simulink model "SEPICPROPELLERLT"  (R2018a)
settings: Solver=ode23  StartTime=0.0  StopTime=11  RelTol=1e-3
undefined symbols (not defined in the file): R, RL
libraries: powerlib x47, powerlib_meascontrol x14, simulink x2
settings Model: Creator=dhanasekar  LastModifiedBy=AVANTHIGHA
settings SolverCC: ZeroCrossAlgorithm=Adaptive
settings DataIOCC: SaveFormat=StructureWithTime  InspectSignalLogs=on
settings OptimizationCC: LifeSpan=inf
settings DebuggingCC: MaxConsecutiveZCsMsg=none  IgnoredZcDiagnostic=none  SFExecutionAtInitializationDiag=none
settings HardwareCC: ProdBitPerSizeT=32  ProdBitPerPtrDiffT=32  ProdWordSize=32  ProdHWDeviceType=Specified
settings CodeAppCC: StateflowObjectComments=on

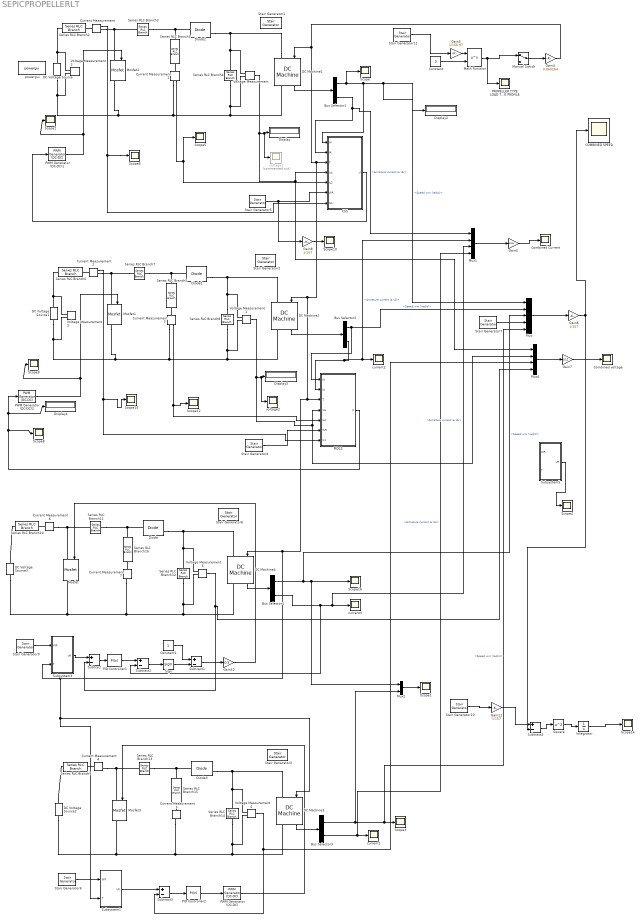
== system SEPICPROPELLERLT ==
  Bus Selector{1..4} (4 alike) : BusSelector  OutputSignals=Speed wm (rad/s),Armature current ia (A)
  COMBINED SPEED : Scope
  CSS : Subsystem
  Combined Current : Scope
  Combined voltage : Scope
  Constant : Constant  Value=3
  Constant1 : Constant
  Current Measurement{,2,4,6} (4 alike) : powerlib/Measurements/Current Measurement  PhasorSimulation=off  OutputType=Complex  PSBequivalent=0
  Current Measurement{1,3,5,7} (4 alike) : powerlib/Measurements/Current Measurement  PhasorSimulation=off  OutputType=Magnitude  PSBequivalent=0
  DC Machine{1..4} (4 alike) : powerlib/Machines/DC Machine  PresetModel=No  MechanicalLoad=Torque TL  FieldType=Permanent magnet  ShowDetailedParameters=on  MeasurementBus=off  RLa="[2.6  0.71285]"  RLf="[ 240  120]"  Laf=1.8  MachineConstant=Back-emf constant (V/rpm)  Ke=0.00525636  Kt=0.05022  J=0.0000886138  Bm=0.000096894  Tf=0  w0=0  Ifinit=1  TsPowergui=0  TsBlock=-1
      settings: SourceProductName=Simscape Electrical
  DC Voltage Source : powerlib/Electrical Sources/DC Voltage Source  Amplitude=6  Measurements=Voltage
  DC Voltage Source1 : powerlib/Electrical Sources/DC Voltage Source  Amplitude=6  Measurements=Voltage
  DC Voltage Source2 : powerlib/Electrical Sources/DC Voltage Source  Amplitude=6  Measurements=Voltage
  DC Voltage Source3 : powerlib/Electrical Sources/DC Voltage Source  Amplitude=7  Measurements=Voltage
  Diode{,1..3} (4 alike) : powerlib/Power Electronics/Diode  Ron=0.001  Lon=0  Vf=0.8  IC=0  UseSnubber=0  Rs=500  Cs=250e-9  Measurements=on
  Display{,2..4} (4 alike) : Display
  Gain10 : Gain  Gain=0.5
  Gain11 : Gain  Gain=1/157
  Gain3 : Gain  Gain=1/156.97
  Gain4 : Gain  Gain=0.060264
  Gain5 : Gain  Gain=1/1.5
  Gain6 : Gain  Gain=1/157
  Gain7 : Gain  Gain=1/12
  Gain8 : Gain  Gain=1/157
  Integrator : Integrator
  Manual Switch : ManualSwitch
  Math Function : Math  Operator=pow  SaturateOnIntegerOverflow=on
  Mosfet{,1..3} (4 alike) : powerlib/Power Electronics/Mosfet  Ron=0.1  Lon=0  Rd=0.01  Vfd=0  IC=0  Rs=1e5  Cs=inf  Measurements=on
      Mosfet1 settings: SourceProductName=Simscape Electrical
      Mosfet2 settings: SourceProductName=Simscape Electrical
  Mux : Mux  Inputs=5
  Mux1 : Mux
  Mux2 : Mux  Inputs=2
  Mux4 : Mux
  PID Controller1 : simulink/Continuous/PID Controller  Controller=PI  TimeDomain=Discrete-time  SampleTime=-1  IntegratorMethod=Forward Euler  FilterMethod=Forward Euler  Form=Parallel  UseFilter=on  ControllerParametersSource=internal  P=0.0009111115  I=1.000777777777777777  D=0.2  N=100  InitialConditionSource=internal  InitialConditionForIntegrator=0  InitialConditionForFilter=0  ExternalReset=none  LimitOutput=off  UpperSaturationLimit=inf  LowerSaturationLimit=-inf  LinearizeAsGain=on  AntiWindupMode=none  Kb=1  TrackingMode=off  Kt=1  PParamMin=[]  PParamMax=[]  IParamMin=[]  IParamMax=[]  DParamMin=[]  DParamMax=[]  NParamMin=[]  NParamMax=[]  KbParamMin=[]  KbParamMax=[]  KtParamMin=[]  KtParamMax=[]  POutMin=[]  POutMax=[]  IOutMin=[]  IOutMax=[]  DOutMin=[]  DOutMax=[]  NOutMin=[]  NOutMax=[]  KbOutMin=[]  KbOutMax=[]  KtOutMin=[]  KtOutMax=[]  IntegratorOutMin=[]  IntegratorOutMax=[]  FilterOutMin=[]  FilterOutMax=[]  SumOutMin=[]  SumOutMax=[]  SumI1OutMin=[]  SumI1OutMax=[]  SumI2OutMin=[]  SumI2OutMax=[]  SumI3OutMin=[]  SumI3OutMax=[]  SumDOutMin=[]  SumDOutMax=[]  SaturationOutMin=[]  SaturationOutMax=[]  IntegratorContinuousStateAttributes=''  IntegratorStateMustResolveToSignalObject=off  IntegratorRTWStateStorageClass=Auto  FilterContinuousStateAttributes=''  FilterStateMustResolveToSignalObject=off  FilterRTWStateStorageClass=Auto  DifferentiatorICPrevScaledInput=0  DifferentiatorOutMin=[]  DifferentiatorOutMax=[]  FilterDiffOutCoefMin=[]  FilterDiffOutCoefMax=[]  SumDenOutMin=[]  SumDenOutMax=[]  SumNumOutMin=[]  SumNumOutMax=[]  ReciprocalOutMin=[]  ReciprocalOutMax=[]  DivideOutMin=[]  DivideOutMax=[]  TunerSelectOption=Transfer Function Based (PID Tuner App)
  PID Controller2 : simulink/Continuous/PID Controller  Controller=PI  TimeDomain=Discrete-time  SampleTime=-1  IntegratorMethod=Forward Euler  FilterMethod=Forward Euler  Form=Parallel  UseFilter=on  ControllerParametersSource=internal  P=0.0000977777777777777777777777777777777777777777777777777777777777777777777777777777111115  I=1.0009999  D=0.2  N=100  InitialConditionSource=internal  InitialConditionForIntegrator=0  InitialConditionForFilter=0  ExternalReset=none  LimitOutput=off  UpperSaturationLimit=inf  LowerSaturationLimit=-inf  LinearizeAsGain=on  AntiWindupMode=none  Kb=1  TrackingMode=off  Kt=1  PParamMin=[]  PParamMax=[]  IParamMin=[]  IParamMax=[]  DParamMin=[]  DParamMax=[]  NParamMin=[]  NParamMax=[]  KbParamMin=[]  KbParamMax=[]  KtParamMin=[]  KtParamMax=[]  POutMin=[]  POutMax=[]  IOutMin=[]  IOutMax=[]  DOutMin=[]  DOutMax=[]  NOutMin=[]  NOutMax=[]  KbOutMin=[]  KbOutMax=[]  KtOutMin=[]  KtOutMax=[]  IntegratorOutMin=[]  IntegratorOutMax=[]  FilterOutMin=[]  FilterOutMax=[]  SumOutMin=[]  SumOutMax=[]  SumI1OutMin=[]  SumI1OutMax=[]  SumI2OutMin=[]  SumI2OutMax=[]  SumI3OutMin=[]  SumI3OutMax=[]  SumDOutMin=[]  SumDOutMax=[]  SaturationOutMin=[]  SaturationOutMax=[]  IntegratorContinuousStateAttributes=''  IntegratorStateMustResolveToSignalObject=off  IntegratorRTWStateStorageClass=Auto  FilterContinuousStateAttributes=''  FilterStateMustResolveToSignalObject=off  FilterRTWStateStorageClass=Auto  DifferentiatorICPrevScaledInput=0  DifferentiatorOutMin=[]  DifferentiatorOutMax=[]  FilterDiffOutCoefMin=[]  FilterDiffOutCoefMax=[]  SumDenOutMin=[]  SumDenOutMax=[]  SumNumOutMin=[]  SumNumOutMax=[]  ReciprocalOutMin=[]  ReciprocalOutMax=[]  DivideOutMin=[]  DivideOutMax=[]  TunerSelectOption=Transfer Function Based (PID Tuner App)
  PIDSS : Subsystem
  PROPELLER TYPE LOAD TORQUE PROFILE : Scope
  PWM Generator (DC-DC) : powerlib_meascontrol/Pulse & Signal Generators/PWM Generator (DC-DC)  Fsw=5000  Ts=0
  PWM Generator (DC-DC)1 : powerlib_meascontrol/Pulse & Signal Generators/PWM Generator (DC-DC)  Fsw=50000  Ts=0
      settings: SourceProductName=Simscape Electrical
  PWM Generator (DC-DC)2 : powerlib_meascontrol/Pulse & Signal Generators/PWM Generator (DC-DC)  Fsw=50000  Ts=0
      settings: SourceProductName=Simscape Electrical
  Scope{,1..6,8..10,12..14,16} (14 alike) : Scope
  Series RLC Branch{1,5..6,15..16} (5 alike) : powerlib/Elements/Series RLC Branch  LConnTagsString=__new0  RConnTagsString=__new0  BranchType=L  Resistance=RL  Inductance=0.5e-3  SetiL0=off  InitialCurrent=0  Capacitance=1e-6  Setx0=off  InitialVoltage=0  Measurements=Branch current
      settings: SourceProductName=Simscape Electrical
  Series RLC Branch10 : powerlib/Elements/Series RLC Branch  LConnTagsString=__new0  RConnTagsString=__new0  BranchType=L  Resistance=RL  Inductance=1e-3  SetiL0=off  InitialCurrent=0  Capacitance=1e-6  Setx0=off  InitialVoltage=0  Measurements=Branch current
      settings: SourceProductName=Simscape Electrical
  Series RLC Branch11 : powerlib/Elements/Series RLC Branch  LConnTagsString=__new0  RConnTagsString=__new0  BranchType=C  Resistance=R  Inductance=1e-3  SetiL0=off  InitialCurrent=0  Capacitance=10000e-6  Setx0=on  InitialVoltage=0  Measurements=Branch voltage
      settings: SourceProductName=Simscape Electrical
  Series RLC Branch{3,7,12..14} (5 alike) : powerlib/Elements/Series RLC Branch  LConnTagsString=__new0  RConnTagsString=__new0  BranchType=C  Resistance=R  Inductance=1e-3  SetiL0=off  InitialCurrent=0  Capacitance=1000e-6  Setx0=on  InitialVoltage=0  Measurements=Branch voltage
      settings: SourceProductName=Simscape Electrical
  Series RLC Branch2 : powerlib/Elements/Series RLC Branch  LConnTagsString=__new0  RConnTagsString=__new0  BranchType=L  Resistance=RL  Inductance=1e-3  SetiL0=off  InitialCurrent=0  Capacitance=1e-6  Setx0=off  InitialVoltage=0  Measurements=Branch current
      settings: SourceProductName=Simscape Electrical
  Series RLC Branch4 : powerlib/Elements/Series RLC Branch  LConnTagsString=__new0  RConnTagsString=__new0  BranchType=C  Resistance=R  Inductance=1e-3  SetiL0=off  InitialCurrent=0  Capacitance=600e-6  Setx0=on  InitialVoltage=0  Measurements=Branch voltage
      settings: SourceProductName=Simscape Electrical
  Series RLC Branch8 : powerlib/Elements/Series RLC Branch  LConnTagsString=__new0  RConnTagsString=__new0  BranchType=C  Resistance=R  Inductance=1e-3  SetiL0=off  InitialCurrent=0  Capacitance=2500e-6  Setx0=on  InitialVoltage=0  Measurements=Branch voltage
      settings: SourceProductName=Simscape Electrical
  Series RLC Branch9 : powerlib/Elements/Series RLC Branch  LConnTagsString=__new0  RConnTagsString=__new0  BranchType=L  Resistance=RL  Inductance=1e-3  SetiL0=off  InitialCurrent=0  Capacitance=1e-6  Setx0=off  InitialVoltage=0  Measurements=Branch current
      settings: SourceProductName=Simscape Electrical
  Sign : Signum
  Square : Math  Operator=square  SaturateOnIntegerOverflow=on
  Stair Generator1 : powerlib_meascontrol/Pulse & Signal Generators/Stair Generator  t=[0,4,8]  e=[0,0.0301,0.0608]  Ts=0
      settings: SourceProductName=Simscape Power Systems
  Stair Generator{4..6,9..11} (6 alike) : powerlib_meascontrol/Pulse & Signal Generators/Stair Generator  t=[0,6,10]  e=[78.5,157,94.2]  Ts=0
      settings: SourceProductName=Simscape Power Systems
  Stair Generator2 : powerlib_meascontrol/Pulse & Signal Generators/Stair Generator  t=[0,4,8]  e=[0,0.0301,0.0602]  Ts=0
      settings: SourceProductName=Simscape Power Systems
  Stair Generator3 : powerlib_meascontrol/Pulse & Signal Generators/Stair Generator  t=[0,4,8]  e=[0,0.0301,0.0602]  Ts=0
      settings: SourceProductName=Simscape Power Systems
  Stair Generator7 : powerlib_meascontrol/Pulse & Signal Generators/Stair Generator  t=[0,6,10]  e=[79.51,158,94.98]  Ts=0
      settings: SourceProductName=Simscape Power Systems
  Stair Generator8 : powerlib_meascontrol/Pulse & Signal Generators/Stair Generator  t=[0,4,8]  e=[0,0.0301,0.0602]  Ts=0
      settings: SourceProductName=Simscape Power Systems
  Subsystem1 : Subsystem
  Subsystem3 : Subsystem
  Subsystem5 : Subsystem
  Subtract{,1..4} (5 alike) : Sum  Inputs=+-
  Voltage Measurement{,1..5} (6 alike) : powerlib/Measurements/Voltage Measurement  PhasorSimulation=off  OutputType=Complex  PSBequivalent=0
  current1 : Scope
  current2 : Scope
  current3 : Scope
  powergui : powerlib/powergui  Priority=1  SimulationMode=Discrete  SampleTime=50e-6  frequency=60  Iterations=50  frequencyindice=0  Pbase=100e6  ErrMax=1e-4  UnitsV=kV  UnitsW=MW  buscounter=0  FunctionMessages=off  echomessages=off  EnableUseOfTLC=off  CurrentSourceSwitches=off  DisableSnubberDevices=off  DisableRonSwitches=off  DisableVfSwitches=off  DisplayEquations=off  SolverType=Tustin/Backward Euler (TBE)  Interpol=off  ExternalGateDelay=off  methode=off  Ts=100  x0status=blocks  SPID=on  SwTol=0  HookPort=off  RestoreLinks=warning  ResistiveCurrentMeasurement=off  Frange=[0:2:500]  Ylog=off  Xlog=on  ShowGrid=off  save=off  variable=ZData  structure=0  ZoomFFT=off  StartTime=0.0  cycles=1  DisplayStyle=1  fundamental=60  FreqAxis=off  MaxFrequency=1000  frequencyindicesteady=1  RmsSteady=1  display=off
  voltage1 : Scope  Commented=on
  voltage2 : Scope
  wires:
  Current Measurement/1 -> CSS/7(IL1), Scope6/1
  Voltage Measurement/1 -> Mux4/1, CSS/4(VA), voltage1/1, Display/1
  Current Measurement1/1 -> CSS/5(IL2), Scope5/1
  PWM Generator (DC-DC)1/1 -> Mosfet2/1, Scope2/1
  DC Machine1/1 -> Bus Selector1/1
  Bus Selector1/1 -> Scope/1, CSS/1(W), Display2/1, Mux/1  "<Speed wm (rad/s)>"
  Bus Selector1/2 -> Mux1/1, CSS/2(IA)  "<Armature current ia (A)>"
  Stair Generator5/1 -> Gain8/1, CSS/6(WR)
  CSS/1(U) -> PWM Generator (DC-DC)1/1
  DC Machine2/1 -> Bus Selector2/1
  Voltage Measurement1/1 -> voltage2/1, Display3/1, Mux4/2, PIDSS/4(VA)
  Bus Selector2/2 -> Mux1/2, current2/1, PIDSS/2(IA)  "<Armature current ia (A)>"
  PIDSS/1(U) -> Scope8/1, Display4/1, PWM Generator (DC-DC)2/1
  Current Measurement2/1 -> Scope13/1, PIDSS/7(IL1)
  Stair Generator4/1 -> PIDSS/6(WR)
  Current Measurement3/1 -> Scope12/1, PIDSS/5(IL2)
  PWM Generator (DC-DC)2/1 -> Mosfet1/1, Scope9/1
  Bus Selector2/1 -> Mux/2, PIDSS/1(W)  "<Speed wm (rad/s)>"
  Gain5/1 -> Combined Current/1
  Mux1/1 -> Gain5/1
  Mux4/1 -> Gain7/1
  Gain7/1 -> Combined voltage/1
  Mux/1 -> Gain6/1
  Gain6/1 -> Subtract4/2, COMBINED SPEED/1
  Stair Generator7/1 -> Mux/4
  Gain8/1 -> Scope10/1
  Voltage Measurement4/1 -> Mux4/3, Subtract3/2
  Integrator/1 -> Scope14/1
  Subtract/1 -> PID Controller1/1
  Square/1 -> Integrator/1
  Subtract3/1 -> PID Controller2/1
  Gain11/1 -> Subtract4/1
  Subsystem3/1(VR) -> Subtract/1
  Gain10/1 -> Mosfet/1
  PID Controller1/1 -> Subtract2/1
  Subtract2/1 -> Sign/1
  Bus Selector4/2 -> Subtract2/2, Mux1/3, current3/1  "<Armature current ia (A)>"
  Sign/1 -> Subtract1/2
  Constant1/1 -> Subtract1/1
  PID Controller2/1 -> PWM Generator (DC-DC)/1
  Bus Selector4/1 -> Mux/3, Mux2/1, Scope16/1  "<Speed wm (rad/s)>"
  Stair Generator6/1 -> Subsystem1/1(WR)
  Subsystem5/1(VR) -> Scope4/1
  Subsystem1/1(VR) -> Subtract3/1
  Mux2/1 -> Scope1/1
  Voltage Measurement5/1 -> Mux4/4, Subtract/2
  PWM Generator (DC-DC)/1 -> Mosfet3/1
  Stair Generator10/1 -> Gain11/1
  Bus Selector3/1 -> Mux2/2, Mux/5, Scope3/1  "<Speed wm (rad/s)>"
  Subtract1/1 -> Gain10/1
  Subtract4/1 -> Square/1
  Bus Selector3/2 -> Mux1/4, current1/1  "<Armature current ia (A)>"
  DC Machine4/1 -> Bus Selector4/1
  Stair Generator9/1 -> Subsystem3/1(WR)
  DC Machine3/1 -> Bus Selector3/1
  Math Function/1 -> PROPELLER TYPE LOAD TORQUE PROFILE/1, Manual Switch/1
  Gain3/1 -> Math Function/1
  Constant/1 -> Math Function/2
  Stair Generator11/1 -> Gain3/1
  Manual Switch/1 -> Gain4/1
  Gain4/1 -> Subsystem1/2(T), DC Machine3/1, Subsystem3/2(T), DC Machine4/1, PIDSS/3(T), DC Machine2/1, CSS/3(T), DC Machine1/1
  connections:
  DC Voltage Source/RConn1 -- Voltage Measurement2/LConn1 -- Series RLC Branch2/LConn1
  Current Measurement/LConn1 -- Series RLC Branch2/RConn1
  Current Measurement/RConn1 -- Mosfet2/LConn1 -- Series RLC Branch3/LConn1
  Series RLC Branch3/RConn1 -- Series RLC Branch1/LConn1 -- Diode2/LConn1
  Current Measurement1/LConn1 -- Series RLC Branch1/RConn1
  DC Machine1/LConn1 -- Diode2/RConn1 -- Voltage Measurement/LConn1 -- Series RLC Branch4/LConn1
  DC Voltage Source/LConn1 -- Voltage Measurement2/LConn2 -- Mosfet2/RConn1 -- Current Measurement1/RConn1 -- Voltage Measurement/LConn2 -- Series RLC Branch4/RConn1 -- DC Machine1/RConn1
  DC Machine2/RConn1 -- Voltage Measurement1/LConn2 -- Series RLC Branch8/RConn1 -- Current Measurement3/RConn1 -- Mosfet1/RConn1 -- DC Voltage Source1/LConn1 -- Voltage Measurement3/LConn2
  Series RLC Branch7/LConn1 -- Current Measurement2/RConn1 -- Mosfet1/LConn1
  Diode1/LConn1 -- Series RLC Branch7/RConn1 -- Series RLC Branch5/LConn1
  Series RLC Branch6/LConn1 -- DC Voltage Source1/RConn1 -- Voltage Measurement3/LConn1
  Series RLC Branch8/LConn1 -- Voltage Measurement1/LConn1 -- DC Machine2/LConn1 -- Diode1/RConn1
  Current Measurement3/LConn1 -- Series RLC Branch5/RConn1
  Current Measurement2/LConn1 -- Series RLC Branch6/RConn1
  Voltage Measurement5/LConn1 -- Series RLC Branch12/LConn1 -- DC Machine4/LConn1 -- Diode/RConn1
  Diode/LConn1 -- Series RLC Branch16/LConn1 -- Series RLC Branch11/RConn1
  Voltage Measurement4/LConn1 -- Series RLC Branch14/LConn1 -- DC Machine3/LConn1 -- Diode3/RConn1
  Mosfet3/LConn1 -- Current Measurement4/RConn1 -- Series RLC Branch13/LConn1
  Mosfet/RConn1 -- DC Voltage Source3/LConn1 -- Current Measurement7/RConn1 -- DC Machine4/RConn1 -- Voltage Measurement5/LConn2 -- Series RLC Branch12/RConn1
  Mosfet/LConn1 -- Current Measurement6/RConn1 -- Series RLC Branch11/LConn1
  Series RLC Branch14/RConn1 -- Current Measurement5/RConn1 -- DC Voltage Source2/LConn1 -- Mosfet3/RConn1 -- DC Machine3/RConn1 -- Voltage Measurement4/LConn2
  Diode3/LConn1 -- Series RLC Branch15/LConn1 -- Series RLC Branch13/RConn1
  Current Measurement7/LConn1 -- Series RLC Branch16/RConn1
  Current Measurement6/LConn1 -- Series RLC Branch10/RConn1
  Current Measurement4/LConn1 -- Series RLC Branch9/RConn1
  DC Voltage Source2/RConn1 -- Series RLC Branch9/LConn1
  Current Measurement5/LConn1 -- Series RLC Branch15/RConn1
  DC Voltage Source3/RConn1 -- Series RLC Branch10/LConn1

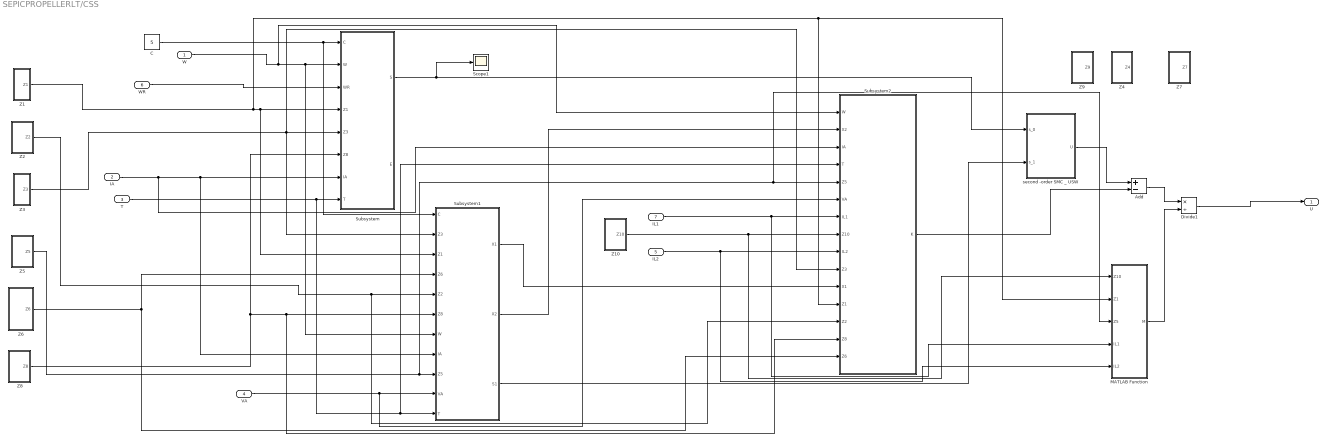
== system SEPICPROPELLERLT/CSS ==
  W : Inport
  IA : Inport  Port=2
  T : Inport  Port=3
  VA : Inport  Port=4
  IL2 : Inport  Port=5
  WR : Inport  Port=6
  IL1 : Inport  Port=7
  Add : Sum  Inputs=+-
  C : Constant  Value=5
  Divide1 : Product  Inputs=*/
  MATLAB Function : MATLAB Function  TreatAsAtomicUnit=on
  Scope1 : Scope
  Subsystem : Subsystem
  Subsystem1 : Subsystem
  Subsystem2 : Subsystem
  Z1 : Subsystem
  Z10 : Subsystem
  Z2 : Subsystem
  Z3 : Subsystem
  Z4 : Subsystem
  Z5 : Subsystem
  Z6 : Subsystem
  Z7 : Subsystem
  Z8 : Subsystem
  Z9 : Subsystem
  second -order SMC _ USW : Subsystem
  U : Outport
  wires:
  C/1 -> Subsystem1/1(C), Subsystem/1(C)
  W/1 -> Subsystem2/1(W), Subsystem1/7(W), Subsystem/2(W)
  WR/1 -> Subsystem/3(WR)
  Z1/1(Z1) -> Subsystem2/12(Z1), MATLAB Function/2(Z1), Subsystem/4(Z1), Subsystem1/3(Z1)
  Z3/1(Z3) -> Subsystem1/2(Z3), Subsystem/5(Z3), Subsystem2/10(Z3)
  Z8/1(Z8) -> Subsystem/6(Z8), Subsystem2/14(Z8), Subsystem1/6(Z8)
  IA/1 -> Subsystem2/3(IA), Subsystem1/8(IA), Subsystem/7(IA)
  T/1 -> Subsystem/8(T), Subsystem2/4(T), Subsystem1/11(T)
  Z6/1(Z6) -> Subsystem2/15(Z6), Subsystem1/4(Z6)
  Z2/1(Z2) -> Subsystem2/13(Z2), Subsystem1/5(Z2)
  Z5/1(Z5) -> MATLAB Function/3(Z5), Subsystem2/5(Z5), Subsystem1/9(Z5)
  VA/1 -> Subsystem2/6(VA), Subsystem1/10(VA)
  Subsystem1/2(X2) -> Subsystem2/2(X2)
  IL1/1 -> MATLAB Function/4(IL1), Subsystem2/7(IL1)
  Z10/1(Z10) -> MATLAB Function/1(Z10), Subsystem2/8(Z10)
  IL2/1 -> Subsystem2/9(IL2), MATLAB Function/5(IL2)
  Subsystem1/1(X1) -> Subsystem2/11(X1)
  Subsystem1/3(S1) -> second -order SMC _ USW/2(s_1)
  second -order SMC _ USW/1(U) -> Add/1
  Subsystem2/1(K) -> Add/2
  Add/1 -> Divide1/1
  MATLAB Function/1(M) -> Divide1/2
  Divide1/1 -> U/1
  Subsystem/1(S) -> Scope1/1, second -order SMC _ USW/1(s_0)

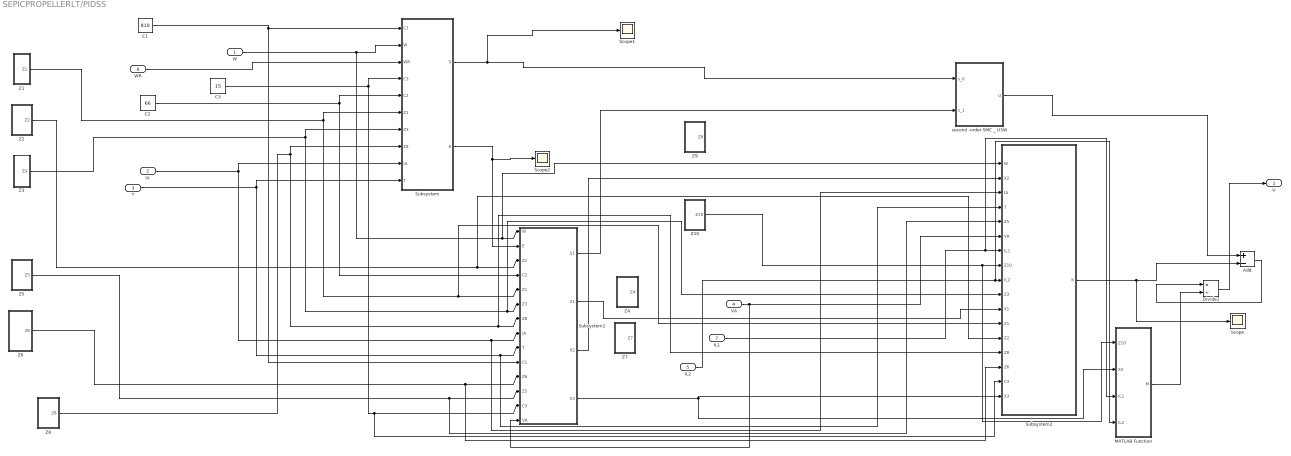
== system SEPICPROPELLERLT/PIDSS ==
  W : Inport
  IA : Inport  Port=2
  T : Inport  Port=3
  VA : Inport  Port=4
  IL2 : Inport  Port=5
  WR : Inport  Port=6
  IL1 : Inport  Port=7
  Add : Sum  Inputs=+-
  C1 : Constant  Value=810
  C2 : Constant  Value=66
  C3 : Constant  Value=15
  Divide1 : Product  Inputs=*/
  MATLAB Function : MATLAB Function  TreatAsAtomicUnit=on
  Scope : Scope
  Scope1 : Scope
  Scope2 : Scope
  Subsystem : Subsystem
  Subsystem1 : Subsystem
  Subsystem2 : Subsystem
  Z1 : Subsystem
  Z10 : Subsystem
  Z2 : Subsystem
  Z3 : Subsystem
  Z4 : Subsystem
  Z5 : Subsystem
  Z6 : Subsystem
  Z7 : Subsystem
  Z8 : Subsystem
  Z9 : Subsystem
  second -order SMC _ USW : Subsystem
  U : Outport
  wires:
  C1/1 -> Subsystem1/10(C1), Subsystem/1(C1)
  W/1 -> Subsystem2/1(W), Subsystem1/1(W), Subsystem/2(W)
  WR/1 -> Subsystem/3(WR)
  C3/1 -> Subsystem/4(C3), Subsystem2/16(C3), Subsystem1/13(C3)
  C2/1 -> Subsystem1/4(C2), Subsystem/5(C2)
  Z1/1(Z1) -> Subsystem2/12(Z1), Subsystem1/5(Z1), Subsystem/6(Z1)
  Z3/1(Z3) -> Subsystem2/10(Z3), Subsystem1/6(Z3), Subsystem/7(Z3)
  Z8/1(Z8) -> Subsystem2/14(Z8), Subsystem1/7(Z8), Subsystem/8(Z8)
  IA/1 -> Subsystem2/3(IA), Subsystem1/8(IA), Subsystem/9(IA)
  T/1 -> Subsystem2/4(T), Subsystem1/9(T), Subsystem/10(T)
  Subsystem/2(E) -> Scope2/1, Subsystem1/2(E)
  Z2/1(Z2) -> Subsystem2/13(Z2), Subsystem1/3(Z2)
  Z6/1(Z6) -> Subsystem2/15(Z6), Subsystem1/11(Z6)
  Z5/1(Z5) -> Subsystem2/5(Z5), Subsystem1/12(Z5)
  Subsystem/1(S) -> second -order SMC _ USW/1(s_0), Scope1/1
  Subsystem1/1(S1) -> second -order SMC _ USW/2(s_1)
  second -order SMC _ USW/1(U) -> Add/1
  Subsystem1/3(X2) -> Subsystem2/2(X2)
  VA/1 -> Subsystem1/14(VA), Subsystem2/6(VA)
  IL1/1 -> MATLAB Function/3(IL1), Subsystem2/7(IL1)
  IL2/1 -> MATLAB Function/4(IL2), Subsystem2/9(IL2)
  Z10/1(Z10) -> MATLAB Function/1(Z10), Subsystem2/8(Z10)
  Subsystem1/2(X1) -> Subsystem2/11(X1)
  Subsystem1/4(X3) -> MATLAB Function/2(X3), Subsystem2/17(X3)
  Subsystem2/1(K) -> Scope/1, Add/2
  Add/1 -> Divide1/1
  MATLAB Function/1(M) -> Divide1/2
  Divide1/1 -> U/1

== system SEPICPROPELLERLT/Subsystem1 ==
  WR : Inport
  T : Inport  Port=2
  A1 : Subsystem
  MATLAB Function : MATLAB Function  TreatAsAtomicUnit=on
  MATLAB Function2 : MATLAB Function  TreatAsAtomicUnit=on
  Subsystem : Subsystem
  Subsystem6 : Subsystem
  VR : Outport
  wires:
  MATLAB Function2/1(VR) -> VR/1
  Subsystem/1(A3) -> MATLAB Function/1(A3)
  A1/1(A1) -> MATLAB Function/5(A1)
  Subsystem6/1(A8) -> MATLAB Function/3(A8)
  MATLAB Function/1(IAS) -> MATLAB Function2/2(IAS)
  WR/1 -> MATLAB Function2/1(WR), MATLAB Function/2(WR)
  T/1 -> MATLAB Function/4(T)

== system SEPICPROPELLERLT/Subsystem3 ==
  WR : Inport
  T : Inport  Port=2
  A1 : Subsystem
  MATLAB Function : MATLAB Function  TreatAsAtomicUnit=on
  MATLAB Function2 : MATLAB Function  TreatAsAtomicUnit=on
  Subsystem : Subsystem
  Subsystem6 : Subsystem
  VR : Outport
  wires:
  MATLAB Function2/1(VR) -> VR/1
  Subsystem/1(A3) -> MATLAB Function/1(A3)
  A1/1(A1) -> MATLAB Function/5(A1)
  Subsystem6/1(A8) -> MATLAB Function/3(A8)
  MATLAB Function/1(IAS) -> MATLAB Function2/2(IAS)
  WR/1 -> MATLAB Function2/1(WR), MATLAB Function/2(WR)
  T/1 -> MATLAB Function/4(T)

== system SEPICPROPELLERLT/Subsystem5 ==
  WR : Inport
  T : Inport  Port=2
  A1 : Subsystem
  MATLAB Function : MATLAB Function  TreatAsAtomicUnit=on
  MATLAB Function2 : MATLAB Function  TreatAsAtomicUnit=on
  Subsystem : Subsystem
  Subsystem6 : Subsystem
  VR : Outport
  wires:
  MATLAB Function2/1(VR) -> VR/1
  Subsystem/1(A3) -> MATLAB Function/1(A3)
  A1/1(A1) -> MATLAB Function/5(A1)
  Subsystem6/1(A8) -> MATLAB Function/3(A8)
  MATLAB Function/1(IAS) -> MATLAB Function2/2(IAS)
  WR/1 -> MATLAB Function2/1(WR), MATLAB Function/2(WR)
  T/1 -> MATLAB Function/4(T)

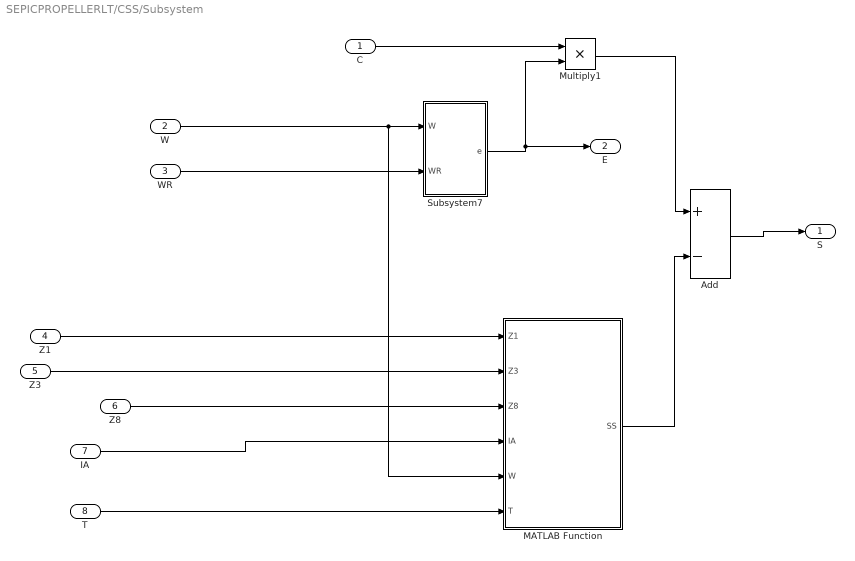
== system SEPICPROPELLERLT/CSS/Subsystem ==
  C : Inport
  W : Inport  Port=2
  WR : Inport  Port=3
  Z1 : Inport  Port=4
  Z3 : Inport  Port=5
  Z8 : Inport  Port=6
  IA : Inport  Port=7
  T : Inport  Port=8
  Add : Sum  Inputs=+-
  MATLAB Function : MATLAB Function  TreatAsAtomicUnit=on
  Multiply1 : Product
  Subsystem7 : Subsystem
  S : Outport
  E : Outport  Port=2
  wires:
  IA/1 -> MATLAB Function/4(IA)
  W/1 -> Subsystem7/1(W), MATLAB Function/5(W)
  Z8/1 -> MATLAB Function/3(Z8)
  MATLAB Function/1(SS) -> Add/2
  Multiply1/1 -> Add/1
  C/1 -> Multiply1/1
  Z1/1 -> MATLAB Function/1(Z1)
  T/1 -> MATLAB Function/6(T)
  Add/1 -> S/1
  WR/1 -> Subsystem7/2(WR)
  Z3/1 -> MATLAB Function/2(Z3)
  Subsystem7/1(e) -> E/1, Multiply1/2

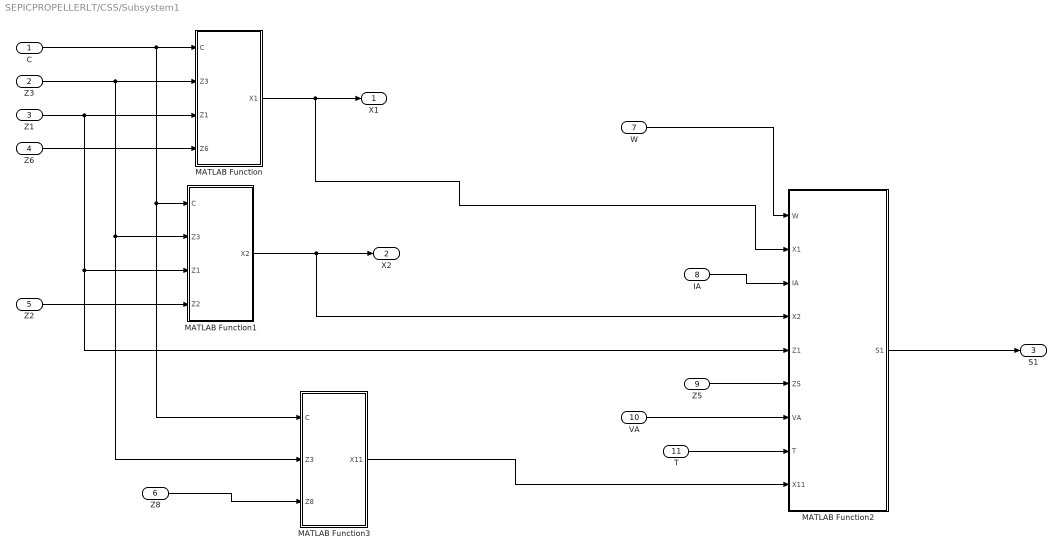
== system SEPICPROPELLERLT/CSS/Subsystem1 ==
  C : Inport
  Z3 : Inport  Port=2
  Z1 : Inport  Port=3
  Z6 : Inport  Port=4
  Z2 : Inport  Port=5
  Z8 : Inport  Port=6
  W : Inport  Port=7
  IA : Inport  Port=8
  Z5 : Inport  Port=9
  VA : Inport  Port=10
  T : Inport  Port=11
  MATLAB Function : MATLAB Function  TreatAsAtomicUnit=on
  MATLAB Function1 : MATLAB Function  TreatAsAtomicUnit=on
  MATLAB Function2 : MATLAB Function  TreatAsAtomicUnit=on
  MATLAB Function3 : MATLAB Function  TreatAsAtomicUnit=on
  X1 : Outport
  X2 : Outport  Port=2
  S1 : Outport  Port=3
  wires:
  MATLAB Function/1(X1) -> MATLAB Function2/2(X1), X1/1
  Z6/1 -> MATLAB Function/4(Z6)
  C/1 -> MATLAB Function3/1(C), MATLAB Function1/1(C), MATLAB Function/1(C)
  Z3/1 -> MATLAB Function3/2(Z3), MATLAB Function1/2(Z3), MATLAB Function/2(Z3)
  MATLAB Function1/1(X2) -> MATLAB Function2/4(X2), X2/1
  Z2/1 -> MATLAB Function1/4(Z2)
  MATLAB Function3/1(X11) -> MATLAB Function2/9(X11)
  Z8/1 -> MATLAB Function3/3(Z8)
  W/1 -> MATLAB Function2/1(W)
  IA/1 -> MATLAB Function2/3(IA)
  Z1/1 -> MATLAB Function2/5(Z1), MATLAB Function1/3(Z1), MATLAB Function/3(Z1)
  Z5/1 -> MATLAB Function2/6(Z5)
  VA/1 -> MATLAB Function2/7(VA)
  T/1 -> MATLAB Function2/8(T)
  MATLAB Function2/1(S1) -> S1/1

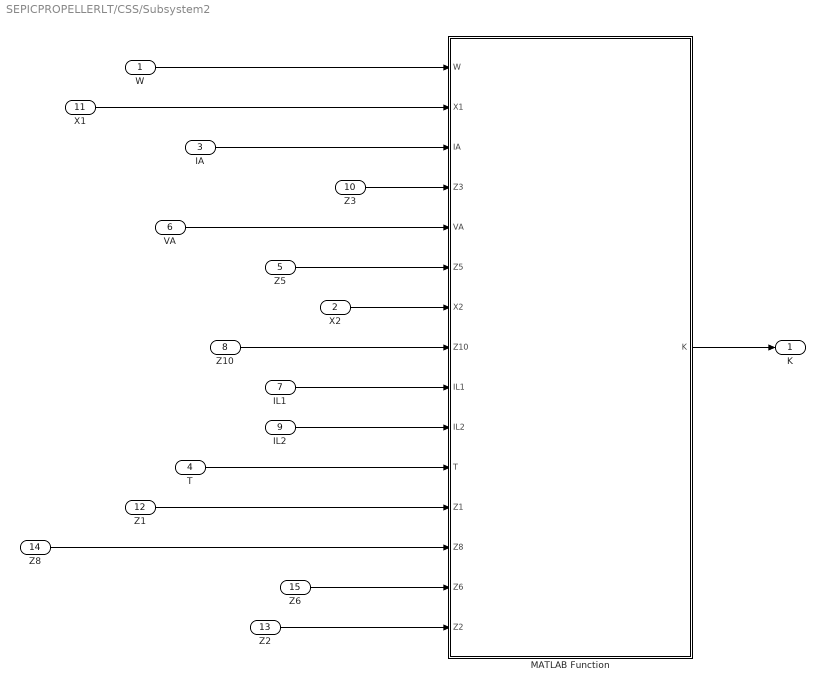
== system SEPICPROPELLERLT/CSS/Subsystem2 ==
  W : Inport
  X2 : Inport  Port=2
  IA : Inport  Port=3
  T : Inport  Port=4
  Z5 : Inport  Port=5
  VA : Inport  Port=6
  IL1 : Inport  Port=7
  Z10 : Inport  Port=8
  IL2 : Inport  Port=9
  Z3 : Inport  Port=10
  X1 : Inport  Port=11
  Z1 : Inport  Port=12
  Z2 : Inport  Port=13
  Z8 : Inport  Port=14
  Z6 : Inport  Port=15
  MATLAB Function : MATLAB Function  TreatAsAtomicUnit=on
  K : Outport
  wires:
  IA/1 -> MATLAB Function/3(IA)
  W/1 -> MATLAB Function/1(W)
  T/1 -> MATLAB Function/11(T)
  X2/1 -> MATLAB Function/7(X2)
  Z5/1 -> MATLAB Function/6(Z5)
  VA/1 -> MATLAB Function/5(VA)
  IL1/1 -> MATLAB Function/9(IL1)
  Z10/1 -> MATLAB Function/8(Z10)
  IL2/1 -> MATLAB Function/10(IL2)
  Z3/1 -> MATLAB Function/4(Z3)
  X1/1 -> MATLAB Function/2(X1)
  Z1/1 -> MATLAB Function/12(Z1)
  Z2/1 -> MATLAB Function/15(Z2)
  Z8/1 -> MATLAB Function/13(Z8)
  Z6/1 -> MATLAB Function/14(Z6)
  MATLAB Function/1(K) -> K/1

== system SEPICPROPELLERLT/CSS/Z1 ==
  Divide : Product  Inputs=*/
  J : Constant  Value=0.0000886138
  KT : Constant  Value=0.05022
  Z1 : Outport
  wires:
  KT/1 -> Divide/1
  Divide/1 -> Z1/1
  J/1 -> Divide/2

== system SEPICPROPELLERLT/CSS/Z10 ==
  1 : Constant
  C2 : Constant  Value=600e-6
  Divide1 : Product  Inputs=*/
  Z10 : Outport
  wires:
  Divide1/1 -> Z10/1
  1/1 -> Divide1/1
  C2/1 -> Divide1/2

== system SEPICPROPELLERLT/CSS/Z2 ==
  Divide : Product  Inputs=*/
  LA : Constant  Value=0.71285
  RA : Constant  Value=2.6
  Z2 : Outport
  wires:
  Divide/1 -> Z2/1
  RA/1 -> Divide/1
  LA/1 -> Divide/2

== system SEPICPROPELLERLT/CSS/Z3 ==
  B : Constant  Value=0.000096894
  Divide : Product  Inputs=*/
  J : Constant  Value=0.0000886138
  Z3 : Outport
  wires:
  B/1 -> Divide/1
  J/1 -> Divide/2
  Divide/1 -> Z3/1

== system SEPICPROPELLERLT/CSS/Z4 ==
  1 : Constant
  Divide1 : Product  Inputs=*/
  L1 : Constant  Value=10e-3
  Z4 : Outport
  wires:
  Divide1/1 -> Z4/1
  1/1 -> Divide1/1
  L1/1 -> Divide1/2

== system SEPICPROPELLERLT/CSS/Z5 ==
  1 : Constant
  Divide1 : Product  Inputs=*/
  LA1 : Constant  Value=0.71285
  Z5 : Outport
  wires:
  Divide1/1 -> Z5/1
  1/1 -> Divide1/1
  LA1/1 -> Divide1/2

== system SEPICPROPELLERLT/CSS/Z6 ==
  Divide : Product  Inputs=*/
  KE : Constant  Value=0.05022
  LA : Constant  Value=0.71285
  Z6 : Outport
  wires:
  LA/1 -> Divide/2
  KE/1 -> Divide/1
  Divide/1 -> Z6/1

== system SEPICPROPELLERLT/CSS/Z7 ==
  1 : Constant
  Divide1 : Product  Inputs=*/
  L2 : Constant  Value=5e-3
  Z7 : Outport
  wires:
  Divide1/1 -> Z7/1
  1/1 -> Divide1/1
  L2/1 -> Divide1/2

== system SEPICPROPELLERLT/CSS/Z8 ==
  1 : Constant
  Divide1 : Product  Inputs=*/
  J : Constant  Value=0.0000886138
  Z8 : Outport
  wires:
  Divide1/1 -> Z8/1
  1/1 -> Divide1/1
  J/1 -> Divide1/2

== system SEPICPROPELLERLT/CSS/Z9 ==
  1 : Constant
  C1 : Constant  Value=10e-6
  Divide1 : Product  Inputs=*/
  Z9 : Outport
  wires:
  Divide1/1 -> Z9/1
  1/1 -> Divide1/1
  C1/1 -> Divide1/2

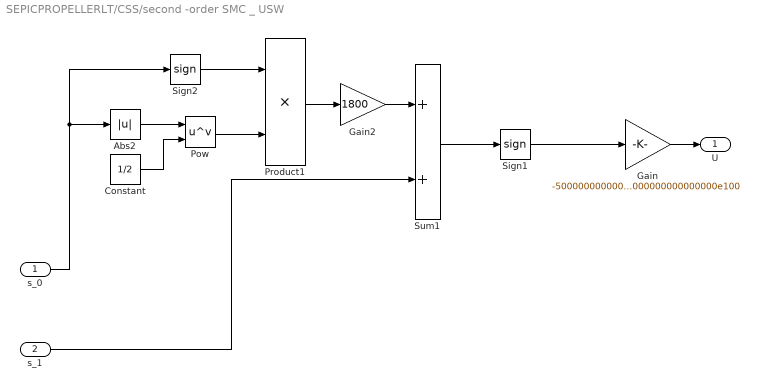
== system SEPICPROPELLERLT/CSS/second -order SMC _ USW ==
  s_0 : Inport
  s_1 : Inport  Port=2
  Abs2 : Abs
  Constant : Constant  Value=1/2
  Gain : Gain  Gain=-500000000000000000000000000000e100
  Gain2 : Gain  Gain=1800
  Pow : Math  Operator=pow  RndMeth=Zero  SaturateOnIntegerOverflow=on
  Product1 : Product
  Sign1 : Signum
  Sign2 : Signum
  Sum1 : Sum
  U : Outport
  wires:
  Gain/1 -> U/1
  s_0/1 -> Sign2/1, Abs2/1
  s_1/1 -> Sum1/2
  Sum1/1 -> Sign1/1
  Gain2/1 -> Sum1/1
  Product1/1 -> Gain2/1
  Abs2/1 -> Pow/1
  Pow/1 -> Product1/2
  Sign2/1 -> Product1/1
  Constant/1 -> Pow/2
  Sign1/1 -> Gain/1

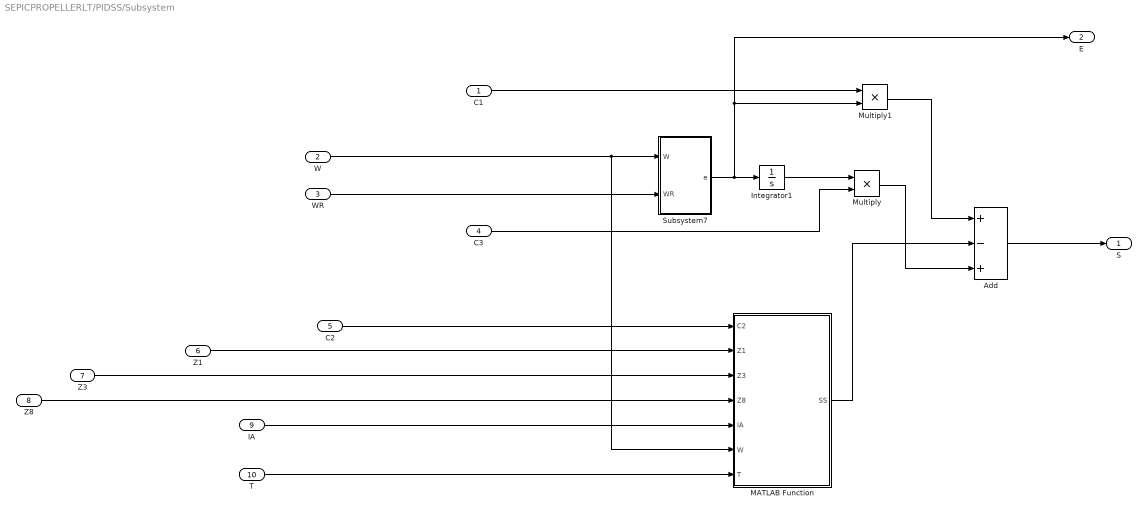
== system SEPICPROPELLERLT/PIDSS/Subsystem ==
  C1 : Inport
  W : Inport  Port=2
  WR : Inport  Port=3
  C3 : Inport  Port=4
  C2 : Inport  Port=5
  Z1 : Inport  Port=6
  Z3 : Inport  Port=7
  Z8 : Inport  Port=8
  IA : Inport  Port=9
  T : Inport  Port=10
  Add : Sum  Inputs=+-+
  Integrator1 : Integrator
  MATLAB Function : MATLAB Function  TreatAsAtomicUnit=on
  Multiply : Product
  Multiply1 : Product
  Subsystem7 : Subsystem
  S : Outport
  E : Outport  Port=2
  wires:
  IA/1 -> MATLAB Function/5(IA)
  W/1 -> MATLAB Function/6(W), Subsystem7/1(W)
  Z8/1 -> MATLAB Function/4(Z8)
  Multiply/1 -> Add/3
  MATLAB Function/1(SS) -> Add/2
  Subsystem7/1(e) -> E/1, Multiply1/2, Integrator1/1
  Multiply1/1 -> Add/1
  C1/1 -> Multiply1/1
  Z1/1 -> MATLAB Function/2(Z1)
  Integrator1/1 -> Multiply/1
  C2/1 -> MATLAB Function/1(C2)
  T/1 -> MATLAB Function/7(T)
  Add/1 -> S/1
  C3/1 -> Multiply/2
  WR/1 -> Subsystem7/2(WR)
  Z3/1 -> MATLAB Function/3(Z3)

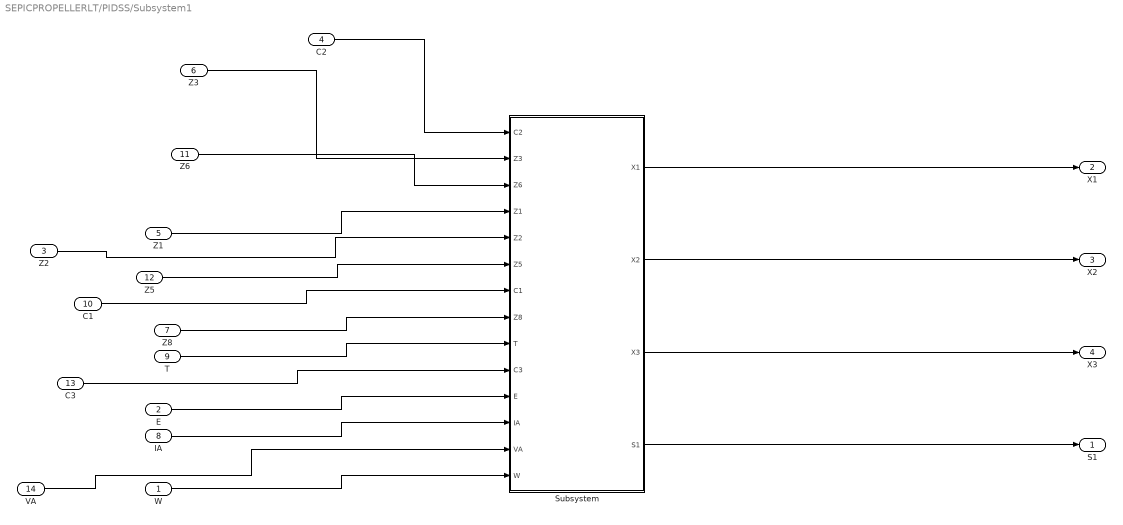
== system SEPICPROPELLERLT/PIDSS/Subsystem1 ==
  W : Inport
  E : Inport  Port=2
  Z2 : Inport  Port=3
  C2 : Inport  Port=4
  Z1 : Inport  Port=5
  Z3 : Inport  Port=6
  Z8 : Inport  Port=7
  IA : Inport  Port=8
  T : Inport  Port=9
  C1 : Inport  Port=10
  Z6 : Inport  Port=11
  Z5 : Inport  Port=12
  C3 : Inport  Port=13
  VA : Inport  Port=14
  Subsystem : Subsystem
  S1 : Outport
  X1 : Outport  Port=2
  X2 : Outport  Port=3
  X3 : Outport  Port=4
  wires:
  Subsystem/4(S1) -> S1/1
  Subsystem/1(X1) -> X1/1
  Subsystem/3(X3) -> X3/1
  Subsystem/2(X2) -> X2/1
  W/1 -> Subsystem/14(W)
  T/1 -> Subsystem/9(T)
  IA/1 -> Subsystem/12(IA)
  E/1 -> Subsystem/11(E)
  C2/1 -> Subsystem/1(C2)
  Z3/1 -> Subsystem/2(Z3)
  Z8/1 -> Subsystem/8(Z8)
  Z1/1 -> Subsystem/4(Z1)
  Z5/1 -> Subsystem/6(Z5)
  Z6/1 -> Subsystem/3(Z6)
  Z2/1 -> Subsystem/5(Z2)
  C1/1 -> Subsystem/7(C1)
  C3/1 -> Subsystem/10(C3)
  VA/1 -> Subsystem/13(VA)

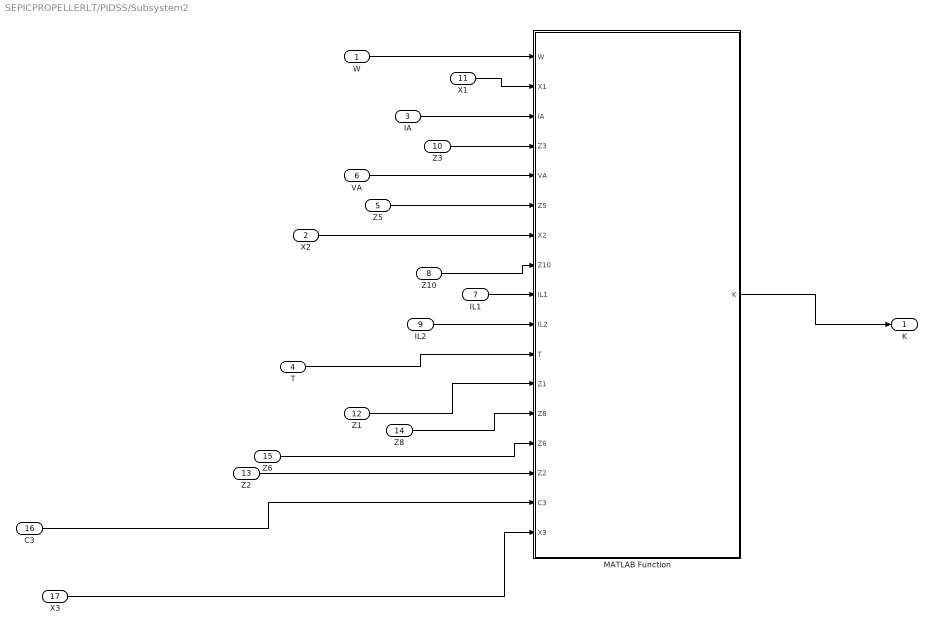
== system SEPICPROPELLERLT/PIDSS/Subsystem2 ==
  W : Inport
  X2 : Inport  Port=2
  IA : Inport  Port=3
  T : Inport  Port=4
  Z5 : Inport  Port=5
  VA : Inport  Port=6
  IL1 : Inport  Port=7
  Z10 : Inport  Port=8
  IL2 : Inport  Port=9
  Z3 : Inport  Port=10
  X1 : Inport  Port=11
  Z1 : Inport  Port=12
  Z2 : Inport  Port=13
  Z8 : Inport  Port=14
  Z6 : Inport  Port=15
  C3 : Inport  Port=16
  X3 : Inport  Port=17
  MATLAB Function : MATLAB Function  TreatAsAtomicUnit=on
  K : Outport
  wires:
  IA/1 -> MATLAB Function/3(IA)
  W/1 -> MATLAB Function/1(W)
  T/1 -> MATLAB Function/11(T)
  X2/1 -> MATLAB Function/7(X2)
  Z5/1 -> MATLAB Function/6(Z5)
  VA/1 -> MATLAB Function/5(VA)
  IL1/1 -> MATLAB Function/9(IL1)
  Z10/1 -> MATLAB Function/8(Z10)
  IL2/1 -> MATLAB Function/10(IL2)
  Z3/1 -> MATLAB Function/4(Z3)
  X1/1 -> MATLAB Function/2(X1)
  Z1/1 -> MATLAB Function/12(Z1)
  Z2/1 -> MATLAB Function/15(Z2)
  Z8/1 -> MATLAB Function/13(Z8)
  Z6/1 -> MATLAB Function/14(Z6)
  C3/1 -> MATLAB Function/16(C3)
  X3/1 -> MATLAB Function/17(X3)
  MATLAB Function/1(K) -> K/1

== system SEPICPROPELLERLT/PIDSS/Z1 ==
  Divide : Product  Inputs=*/
  J : Constant  Value=0.0000886138
  KT : Constant  Value=0.05022
  Z1 : Outport
  wires:
  KT/1 -> Divide/1
  Divide/1 -> Z1/1
  J/1 -> Divide/2

== system SEPICPROPELLERLT/PIDSS/Z10 ==
  1 : Constant
  C2 : Constant  Value=2500e-6
  Divide1 : Product  Inputs=*/
  Z10 : Outport
  wires:
  Divide1/1 -> Z10/1
  1/1 -> Divide1/1
  C2/1 -> Divide1/2

== system SEPICPROPELLERLT/PIDSS/Z2 ==
  Divide : Product  Inputs=*/
  LA : Constant  Value=0.71285
  RA : Constant  Value=2.6
  Z2 : Outport
  wires:
  Divide/1 -> Z2/1
  RA/1 -> Divide/1
  LA/1 -> Divide/2

== system SEPICPROPELLERLT/PIDSS/Z3 ==
  B : Constant  Value=0.000096894
  Divide : Product  Inputs=*/
  J : Constant  Value=0.0000886138
  Z3 : Outport
  wires:
  B/1 -> Divide/1
  J/1 -> Divide/2
  Divide/1 -> Z3/1

== system SEPICPROPELLERLT/PIDSS/Z4 ==
  1 : Constant
  Divide1 : Product  Inputs=*/
  L1 : Constant  Value=10e-3
  Z4 : Outport
  wires:
  Divide1/1 -> Z4/1
  1/1 -> Divide1/1
  L1/1 -> Divide1/2

== system SEPICPROPELLERLT/PIDSS/Z5 ==
  1 : Constant
  Divide1 : Product  Inputs=*/
  LA1 : Constant  Value=0.71285
  Z5 : Outport
  wires:
  Divide1/1 -> Z5/1
  1/1 -> Divide1/1
  LA1/1 -> Divide1/2

== system SEPICPROPELLERLT/PIDSS/Z6 ==
  Divide : Product  Inputs=*/
  KE : Constant  Value=0.05022
  LA : Constant  Value=0.71285
  Z6 : Outport
  wires:
  LA/1 -> Divide/2
  KE/1 -> Divide/1
  Divide/1 -> Z6/1

== system SEPICPROPELLERLT/PIDSS/Z7 ==
  1 : Constant
  Divide1 : Product  Inputs=*/
  L2 : Constant  Value=5e-3
  Z7 : Outport
  wires:
  Divide1/1 -> Z7/1
  1/1 -> Divide1/1
  L2/1 -> Divide1/2

== system SEPICPROPELLERLT/PIDSS/Z8 ==
  1 : Constant
  Divide1 : Product  Inputs=*/
  J : Constant  Value=0.0000886138
  Z8 : Outport
  wires:
  Divide1/1 -> Z8/1
  1/1 -> Divide1/1
  J/1 -> Divide1/2

== system SEPICPROPELLERLT/PIDSS/Z9 ==
  1 : Constant
  C1 : Constant  Value=10e-6
  Divide1 : Product  Inputs=*/
  Z9 : Outport
  wires:
  Divide1/1 -> Z9/1
  1/1 -> Divide1/1
  C1/1 -> Divide1/2

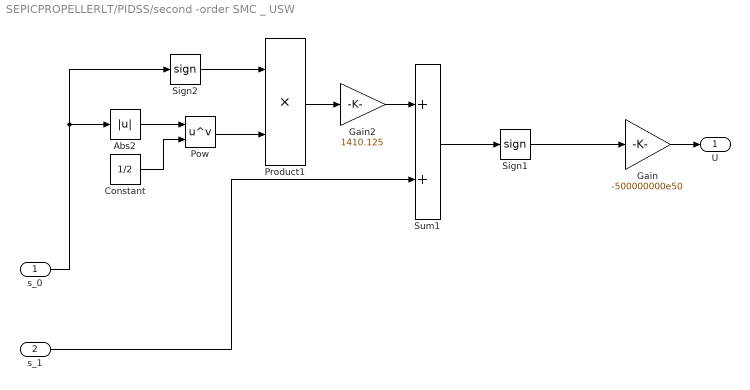
== system SEPICPROPELLERLT/PIDSS/second -order SMC _ USW ==
  s_0 : Inport
  s_1 : Inport  Port=2
  Abs2 : Abs
  Constant : Constant  Value=1/2
  Gain : Gain  Gain=-500000000e50
  Gain2 : Gain  Gain=1410.125
  Pow : Math  Operator=pow  RndMeth=Zero  SaturateOnIntegerOverflow=on
  Product1 : Product
  Sign1 : Signum
  Sign2 : Signum
  Sum1 : Sum
  U : Outport
  wires:
  Gain/1 -> U/1
  s_0/1 -> Sign2/1, Abs2/1
  s_1/1 -> Sum1/2
  Sum1/1 -> Sign1/1
  Gain2/1 -> Sum1/1
  Product1/1 -> Gain2/1
  Abs2/1 -> Pow/1
  Pow/1 -> Product1/2
  Sign2/1 -> Product1/1
  Constant/1 -> Pow/2
  Sign1/1 -> Gain/1

== system SEPICPROPELLERLT/Subsystem1/A1 ==
  Divide : Product  Inputs=*/
  J : Constant  Value=0.0000886138
  KT : Constant  Value=0.05022
  A1 : Outport
  wires:
  KT/1 -> Divide/1
  Divide/1 -> A1/1
  J/1 -> Divide/2

== system SEPICPROPELLERLT/Subsystem1/Subsystem ==
  B : Constant  Value=0.000096894
  Divide : Product  Inputs=*/
  J : Constant  Value=0.0000886138
  A3 : Outport
  wires:
  B/1 -> Divide/1
  J/1 -> Divide/2
  Divide/1 -> A3/1

== system SEPICPROPELLERLT/Subsystem1/Subsystem6 ==
  1 : Constant
  Divide1 : Product  Inputs=*/
  J : Constant  Value=0.0000886138
  A8 : Outport
  wires:
  Divide1/1 -> A8/1
  1/1 -> Divide1/1
  J/1 -> Divide1/2

== system SEPICPROPELLERLT/Subsystem3/A1 ==
  Divide : Product  Inputs=*/
  J : Constant  Value=0.0000886138
  KT : Constant  Value=0.05022
  A1 : Outport
  wires:
  KT/1 -> Divide/1
  Divide/1 -> A1/1
  J/1 -> Divide/2

== system SEPICPROPELLERLT/Subsystem3/Subsystem ==
  B : Constant  Value=0.000096894
  Divide : Product  Inputs=*/
  J : Constant  Value=0.0000886138
  A3 : Outport
  wires:
  B/1 -> Divide/1
  J/1 -> Divide/2
  Divide/1 -> A3/1

== system SEPICPROPELLERLT/Subsystem3/Subsystem6 ==
  1 : Constant
  Divide1 : Product  Inputs=*/
  J : Constant  Value=0.0000886138
  A8 : Outport
  wires:
  Divide1/1 -> A8/1
  1/1 -> Divide1/1
  J/1 -> Divide1/2

== system SEPICPROPELLERLT/Subsystem5/A1 ==
  Divide : Product  Inputs=*/
  J : Constant  Value=0.0000886138
  KT : Constant  Value=0.05022
  A1 : Outport
  wires:
  KT/1 -> Divide/1
  Divide/1 -> A1/1
  J/1 -> Divide/2

== system SEPICPROPELLERLT/Subsystem5/Subsystem ==
  B : Constant  Value=0.000096894
  Divide : Product  Inputs=*/
  J : Constant  Value=0.0000886138
  A3 : Outport
  wires:
  B/1 -> Divide/1
  J/1 -> Divide/2
  Divide/1 -> A3/1

== system SEPICPROPELLERLT/Subsystem5/Subsystem6 ==
  1 : Constant
  Divide1 : Product  Inputs=*/
  J : Constant  Value=0.0000886138
  A8 : Outport
  wires:
  Divide1/1 -> A8/1
  1/1 -> Divide1/1
  J/1 -> Divide1/2

== system SEPICPROPELLERLT/CSS/Subsystem/Subsystem7 ==
  W : Inport
  WR : Inport  Port=2
  MATLAB Function : MATLAB Function  TreatAsAtomicUnit=on
  e : Outport
  wires:
  MATLAB Function/1(e) -> e/1
  W/1 -> MATLAB Function/2(W)
  WR/1 -> MATLAB Function/1(WR)

== system SEPICPROPELLERLT/PIDSS/Subsystem/Subsystem7 ==
  W : Inport
  WR : Inport  Port=2
  MATLAB Function : MATLAB Function  TreatAsAtomicUnit=on
  e : Outport
  wires:
  MATLAB Function/1(e) -> e/1
  W/1 -> MATLAB Function/2(W)
  WR/1 -> MATLAB Function/1(WR)

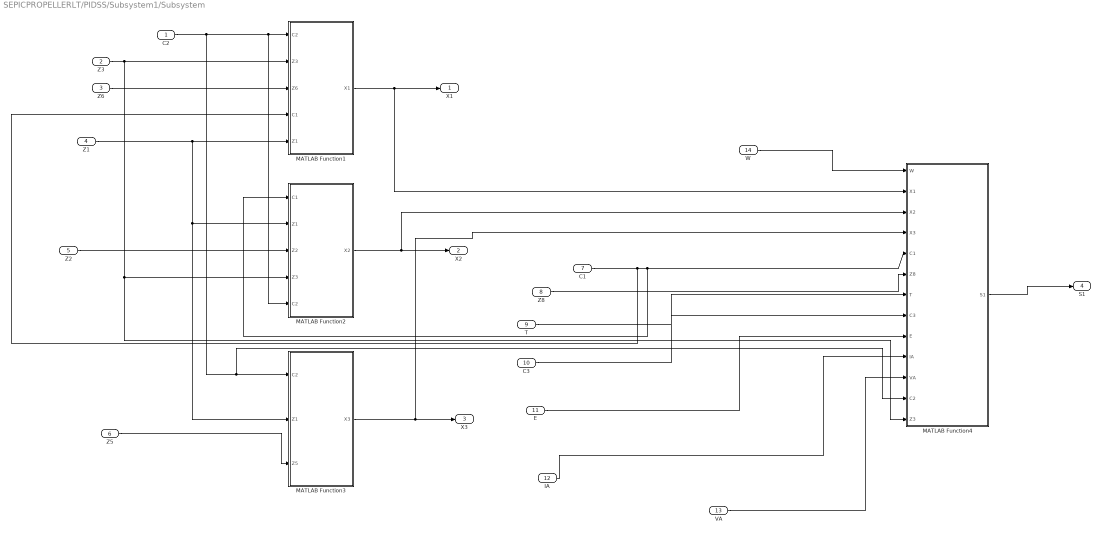
== system SEPICPROPELLERLT/PIDSS/Subsystem1/Subsystem ==
  C2 : Inport
  Z3 : Inport  Port=2
  Z6 : Inport  Port=3
  Z1 : Inport  Port=4
  Z2 : Inport  Port=5
  Z5 : Inport  Port=6
  C1 : Inport  Port=7
  Z8 : Inport  Port=8
  T : Inport  Port=9
  C3 : Inport  Port=10
  E : Inport  Port=11
  IA : Inport  Port=12
  VA : Inport  Port=13
  W : Inport  Port=14
  MATLAB Function1 : MATLAB Function  TreatAsAtomicUnit=on
  MATLAB Function2 : MATLAB Function  TreatAsAtomicUnit=on
  MATLAB Function3 : MATLAB Function  TreatAsAtomicUnit=on
  MATLAB Function4 : MATLAB Function  TreatAsAtomicUnit=on
  X1 : Outport
  X2 : Outport  Port=2
  X3 : Outport  Port=3
  S1 : Outport  Port=4
  wires:
  MATLAB Function2/1(X2) -> MATLAB Function4/3(X2), X2/1
  Z5/1 -> MATLAB Function3/3(Z5)
  C2/1 -> MATLAB Function4/12(C2), MATLAB Function3/1(C2), MATLAB Function2/5(C2), MATLAB Function1/1(C2)
  MATLAB Function3/1(X3) -> MATLAB Function4/4(X3), X3/1
  Z1/1 -> MATLAB Function2/2(Z1), MATLAB Function3/2(Z1), MATLAB Function1/5(Z1)
  Z3/1 -> MATLAB Function4/13(Z3), MATLAB Function2/4(Z3), MATLAB Function1/2(Z3)
  Z2/1 -> MATLAB Function2/3(Z2)
  Z6/1 -> MATLAB Function1/3(Z6)
  C1/1 -> MATLAB Function1/4(C1), MATLAB Function2/1(C1), MATLAB Function4/5(C1)
  MATLAB Function1/1(X1) -> MATLAB Function4/2(X1), X1/1
  Z8/1 -> MATLAB Function4/6(Z8)
  T/1 -> MATLAB Function4/7(T)
  C3/1 -> MATLAB Function4/8(C3)
  E/1 -> MATLAB Function4/9(E)
  IA/1 -> MATLAB Function4/10(IA)
  VA/1 -> MATLAB Function4/11(VA)
  MATLAB Function4/1(S1) -> S1/1
  W/1 -> MATLAB Function4/1(W)

== matlab function SEPICPROPELLERLT/CSS/Subsystem/Subsystem7/MATLAB Function ==
  data: e output; WR input; W input
function e = fcn(WR,W)

e = (WR-W);

== matlab function SEPICPROPELLERLT/CSS/Subsystem/MATLAB Function ==
  data: SS output; Z1 input; Z3 input; Z8 input; IA input; W input; T input
function SS = fcn(Z1,Z3,Z8,IA,W,T)

SS = ((Z1*IA)-(Z3*W)-(Z8*T));

== matlab function SEPICPROPELLERLT/CSS/Subsystem1/MATLAB Function ==
  data: C input; X1 output; Z3 input; Z1 input; Z6 input
function X1 = fcn(C,Z3,Z1,Z6)

X1 = ((C*Z3)+(Z1*Z6)-(Z3*Z3));

== matlab function SEPICPROPELLERLT/CSS/Subsystem1/MATLAB Function1 ==
  data: C input; X2 output; Z3 input; Z1 input; Z2 input
function X2 = fcn(C,Z3,Z1,Z2)

X2 = ((Z1*Z2)-(C*Z1)+(Z3*Z1));

== matlab function SEPICPROPELLERLT/CSS/Subsystem1/MATLAB Function2 ==
  data: W input; S1 output; X1 input; IA input; X2 input; Z1 input; Z5 input; VA input; T input; X11 input
function S1 = fcn(W,X1,IA,X2,Z1,Z5,VA,T,X11)

S1 = ((W*X1)+(IA*X2)-(Z1*Z5*VA)+(T*X11));

== matlab function SEPICPROPELLERLT/CSS/Subsystem1/MATLAB Function3 ==
  data: C input; X11 output; Z3 input; Z8 input
function X11 = fcn(C,Z3,Z8)

X11 = ((C*Z8)-(Z3*Z8));

== matlab function SEPICPROPELLERLT/CSS/Subsystem2/MATLAB Function ==
  data: W input; X1 input; IA input; Z3 input; VA input; Z5 input; X2 input; Z10 input; IL1 input; IL2 input; T input; K output; Z1 input; Z8 input; Z6 input; Z2 input
function K = fcn(W,X1,IA,Z3,VA,Z5,X2,Z10,IL1,IL2,T,Z1,Z8,Z6,Z2)

K = ((Z1*IA*X1)-(Z3*W*X1)-(Z8*T*X1)-(Z6*W*X2)-(Z2*IA*X2)+(Z5*VA*X2)-(IL1*Z1*Z5*Z10)-(IL2*Z1*Z5*Z10)+(Z10*IA*Z1*Z5));

== matlab function SEPICPROPELLERLT/CSS/MATLAB Function ==
  data: Z10 input; M output; Z1 input; Z5 input; IL1 input; IL2 input
function M = fcn(Z10,Z1,Z5,IL1,IL2)

M = ((Z10*Z1*Z5*(IL1+IL2)));

== matlab function SEPICPROPELLERLT/PIDSS/MATLAB Function ==
  data: Z10 input; M output; X3 input; IL1 input; IL2 input
function M = fcn(Z10,X3,IL1,IL2)

M = (-(Z10*X3*(IL1+IL2)));

== matlab function SEPICPROPELLERLT/PIDSS/Subsystem/MATLAB Function ==
  data: C2 input; SS output; Z1 input; Z3 input; Z8 input; IA input; W input; T input
function SS = fcn(C2,Z1,Z3,Z8,IA,W,T)

SS = (C2*((Z1*IA)-(Z3*W)-(Z8*T)));

== matlab function SEPICPROPELLERLT/PIDSS/Subsystem/Subsystem7/MATLAB Function ==
  data: e output; WR input; W input
function e = fcn(WR,W)

e = (WR-W);

== matlab function SEPICPROPELLERLT/PIDSS/Subsystem1/Subsystem/MATLAB Function1 ==
  data: X1 output; C2 input; Z3 input; Z6 input; C1 input; Z1 input
function X1 = fcn(C2,Z3,Z6,C1,Z1)

X1 = ((C1*Z3)-(C2*Z3*Z3)+(C2*Z1*Z6));

== matlab function SEPICPROPELLERLT/PIDSS/Subsystem1/Subsystem/MATLAB Function2 ==
  data: X2 output; C1 input; Z1 input; Z2 input; Z3 input; C2 input
function X2 = fcn(C1,Z1,Z2,Z3,C2)

X2 = ((C2*Z1*Z2)-(C1*Z1)+(C2*Z1*Z3));

== matlab function SEPICPROPELLERLT/PIDSS/Subsystem1/Subsystem/MATLAB Function3 ==
  data: X3 output; C2 input; Z1 input; Z5 input
function X3 = fcn(C2,Z1,Z5)

X3 = (-(C2*Z1*Z5));

== matlab function SEPICPROPELLERLT/PIDSS/Subsystem1/Subsystem/MATLAB Function4 ==
  data: S1 output; W input; X1 input; X2 input; X3 input; C1 input; Z8 input; T input; C3 input; E input; IA input; VA input; C2 input; Z3 input
function S1 = fcn(W,X1,X2,X3,C1,Z8,T,C3,E,IA,VA,C2,Z3)

S1 = ((W*X1)+(IA*X2)+(VA*X3)+(C1*Z8*T)+(C3*E)-(C2*Z3*Z8*T));

== matlab function SEPICPROPELLERLT/PIDSS/Subsystem2/MATLAB Function ==
  data: W input; X1 input; IA input; Z3 input; VA input; Z5 input; X2 input; Z10 input; IL1 input; IL2 input; T input; K output; Z1 input; Z8 input; Z6 input; Z2 input; C3 input; X3 input
function K = fcn(W,X1,IA,Z3,VA,Z5,X2,Z10,IL1,IL2,T,Z1,Z8,Z6,Z2,C3,X3)

K = ((Z1*IA*X1)-(Z3*W*X1)-(Z8*T*X1)-(Z6*W*X2)-(Z2*IA*X2)+(Z5*VA*X2)+(Z3*C3*W)-(C3*Z1*IA)+(C3*Z8*T)+(IL1*Z10*X3)+(IL2*Z10*X3)-(Z10*IA*X3));

== matlab function SEPICPROPELLERLT/Subsystem1/MATLAB Function ==
  data: A3 input; IAS output; WR input; A8 input; T input; A1 input
function IAS = fcn(A3,WR,A8,T,A1)

IAS = ((A3*WR)+(A8*T))/A1;

== matlab function SEPICPROPELLERLT/Subsystem1/MATLAB Function2 ==
  data: WR input; VR output; IAS input
function VR = fcn(WR,IAS)

VR = ((0.05022*WR)+(IAS*2.6));

== matlab function SEPICPROPELLERLT/Subsystem3/MATLAB Function ==
  data: A3 input; IAS output; WR input; A8 input; T input; A1 input
function IAS = fcn(A3,WR,A8,T,A1)

IAS = ((A3*WR)+(A8*T))/A1;

== matlab function SEPICPROPELLERLT/Subsystem3/MATLAB Function2 ==
  data: WR input; VR output; IAS input
function VR = fcn(WR,IAS)

VR = ((0.05022*WR)+(IAS*2.6));

== matlab function SEPICPROPELLERLT/Subsystem5/MATLAB Function2 ==
  data: WR input; VR output; IAS input
function VR = fcn(WR,IAS)

VR = ((0.05022*WR)+(IAS*2.6));

== matlab function SEPICPROPELLERLT/Subsystem5/MATLAB Function ==
  data: A3 input; IAS output; WR input; A8 input; T input; A1 input
function IAS = fcn(A3,WR,A8,T,A1)

IAS = ((A3*WR)+(A8*T))/A1;
